simulink model "midProj"  (R2019b)
settings: Solver=VariableStepAuto  StartTime=0.0  StopTime=8  RelTol=1e-3
values from neighbouring files (symbols this model uses):
  X = 1    [midProj1102.m]    (also in midProj1103.m)
  Y = 1    [midProj1102.m]    (also in midProj1103.m)
undefined symbols (not defined in the file or in its folder): PhiDesire, PhoDesire
libraries: simulink x3
settings Model: Creator=yuhaiyang  LastModifiedBy=yuhaiyang

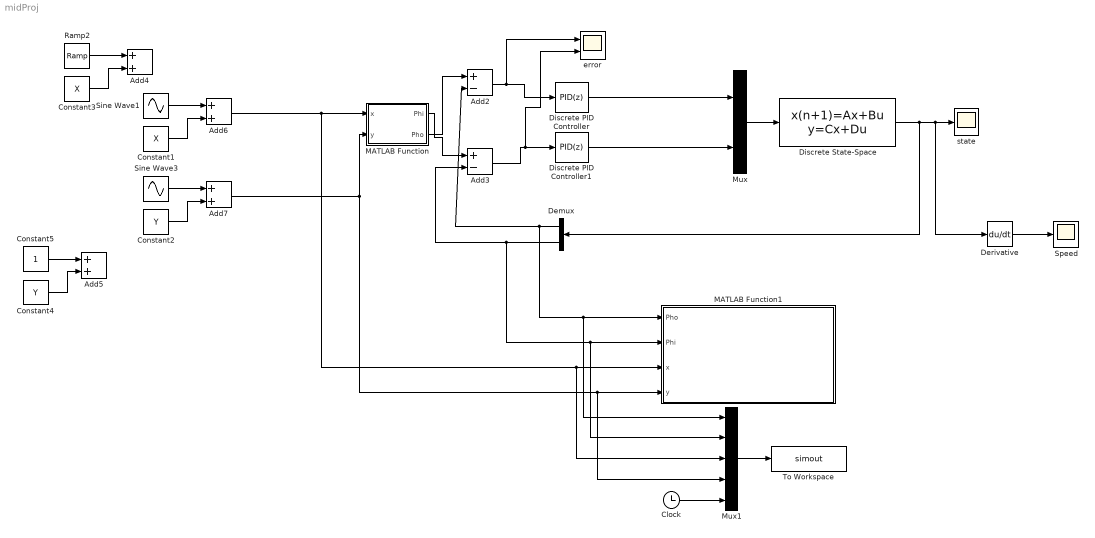
== system midProj ==
  Add2 : Sum  Inputs=+-
  Add3 : Sum  Inputs=+-
  Add{4..7} (4 alike) : Sum
  Clock : Clock
  Constant1 : Constant  Value=X
  Constant2 : Constant  Value=Y
  Constant3 : Constant  Value=X
  Constant4 : Constant  Value=Y
  Constant5 : Constant
  Demux : Demux  Outputs=2
  Derivative : Derivative
  Discrete PID Controller : simulink/Continuous/PID Controller  Controller=PID  Form=Parallel  TimeDomain=Discrete-time  SampleTime=step  IntegratorMethod=Forward Euler  FilterMethod=Forward Euler  ControllerParametersSource=internal  P=0.0451594253248729  I=0.00606949033779435  D=0.0825217736897104  UseFilter=on  N=17.4747024685303  TunerSelectOption=Transfer Function Based (PID Tuner App)  InitialConditionSource=internal  InitialConditionForIntegrator=0  InitialConditionForFilter=0  DifferentiatorICPrevScaledInput=0  ExternalReset=none  TrackingMode=off  Kt=1  LimitOutput=off  UpperSaturationLimit=inf  LowerSaturationLimit=-inf  LinearizeAsGain=off  AntiWindupMode=none  Kb=1  POutMin=[]  POutMax=[]  IOutMin=[]  IOutMax=[]  DOutMin=[]  DOutMax=[]  NOutMin=[]  NOutMax=[]  SumOutMin=[]  SumOutMax=[]  SaturationOutMin=[]  SaturationOutMax=[]  PParamMin=[]  PParamMax=[]  IParamMin=[]  IParamMax=[]  DParamMin=[]  DParamMax=[]  NParamMin=[]  NParamMax=[]  KbParamMin=[]  KbParamMax=[]  KtParamMin=[]  KtParamMax=[]  KbOutMin=[]  KbOutMax=[]  KtOutMin=[]  KtOutMax=[]  IntegratorOutMin=[]  IntegratorOutMax=[]  FilterOutMin=[]  FilterOutMax=[]  SumI1OutMin=[]  SumI1OutMax=[]  SumI2OutMin=[]  SumI2OutMax=[]  SumI3OutMin=[]  SumI3OutMax=[]  SumI4OutMin=[]  SumI4OutMax=[]  SumDOutMin=[]  SumDOutMax=[]  DifferentiatorOutMin=[]  DifferentiatorOutMax=[]  FilterDiffOutCoefMin=[]  FilterDiffOutCoefMax=[]  ReciprocalOutMin=[]  ReciprocalOutMax=[]  SumDenOutMin=[]  SumDenOutMax=[]  SumNumOutMin=[]  SumNumOutMax=[]  DivideOutMin=[]  DivideOutMax=[]  IntegratorContinuousStateAttributes=''  IntegratorStateMustResolveToSignalObject=off  IntegratorRTWStateStorageClass=Auto  FilterContinuousStateAttributes=''  FilterStateMustResolveToSignalObject=off  FilterRTWStateStorageClass=Auto  ParallelPVariant=InternalParameters  IdealPVariant=Disabled  IVariant=InternalParameters  DVariant=InternalParameters  IntegratorVariant=Discrete  SatVariant=Disabled  AWVariant=Passthrough  PCopyVariant=Disabled  TRVariant=Disabled  FdbkBlocksVariant=Forward  IdealPFdbkVariant=Disabled  SatFdbkVariant=Disabled  DerivativeFilterVariant=ForwardEulerFilter  NVariant=InternalParameters  NCopyVariant=Disabled  FilterICVariant=InternalICsFilter  IntegratorICVariant=InternalICs  ExternalResetVariant=Disabled  TRSumVariant=Passthrough  SumFdbkVariant=Disabled  SumVariant=Sum_PID
  Discrete PID Controller1 : simulink/Continuous/PID Controller  Controller=PID  Form=Parallel  TimeDomain=Discrete-time  SampleTime=step  IntegratorMethod=Forward Euler  FilterMethod=Forward Euler  ControllerParametersSource=internal  P=0.0143220434066502  I=0.00109223482739123  D=0.0463013739503765  UseFilter=on  N=12.1025626011462  TunerSelectOption=Transfer Function Based (PID Tuner App)  InitialConditionSource=internal  InitialConditionForIntegrator=0  InitialConditionForFilter=0  DifferentiatorICPrevScaledInput=0  ExternalReset=none  TrackingMode=off  Kt=1  LimitOutput=off  UpperSaturationLimit=inf  LowerSaturationLimit=-inf  LinearizeAsGain=off  AntiWindupMode=none  Kb=1  POutMin=[]  POutMax=[]  IOutMin=[]  IOutMax=[]  DOutMin=[]  DOutMax=[]  NOutMin=[]  NOutMax=[]  SumOutMin=[]  SumOutMax=[]  SaturationOutMin=[]  SaturationOutMax=[]  PParamMin=[]  PParamMax=[]  IParamMin=[]  IParamMax=[]  DParamMin=[]  DParamMax=[]  NParamMin=[]  NParamMax=[]  KbParamMin=[]  KbParamMax=[]  KtParamMin=[]  KtParamMax=[]  KbOutMin=[]  KbOutMax=[]  KtOutMin=[]  KtOutMax=[]  IntegratorOutMin=[]  IntegratorOutMax=[]  FilterOutMin=[]  FilterOutMax=[]  SumI1OutMin=[]  SumI1OutMax=[]  SumI2OutMin=[]  SumI2OutMax=[]  SumI3OutMin=[]  SumI3OutMax=[]  SumI4OutMin=[]  SumI4OutMax=[]  SumDOutMin=[]  SumDOutMax=[]  DifferentiatorOutMin=[]  DifferentiatorOutMax=[]  FilterDiffOutCoefMin=[]  FilterDiffOutCoefMax=[]  ReciprocalOutMin=[]  ReciprocalOutMax=[]  SumDenOutMin=[]  SumDenOutMax=[]  SumNumOutMin=[]  SumNumOutMax=[]  DivideOutMin=[]  DivideOutMax=[]  IntegratorContinuousStateAttributes=''  IntegratorStateMustResolveToSignalObject=off  IntegratorRTWStateStorageClass=Auto  FilterContinuousStateAttributes=''  FilterStateMustResolveToSignalObject=off  FilterRTWStateStorageClass=Auto  ParallelPVariant=InternalParameters  IdealPVariant=Disabled  IVariant=InternalParameters  DVariant=InternalParameters  IntegratorVariant=Discrete  SatVariant=Disabled  AWVariant=Passthrough  PCopyVariant=Disabled  TRVariant=Disabled  FdbkBlocksVariant=Forward  IdealPFdbkVariant=Disabled  SatFdbkVariant=Disabled  DerivativeFilterVariant=ForwardEulerFilter  NVariant=InternalParameters  NCopyVariant=Disabled  FilterICVariant=InternalICsFilter  IntegratorICVariant=InternalICs  ExternalResetVariant=Disabled  TRSumVariant=Passthrough  SumFdbkVariant=Disabled  SumVariant=Sum_PID
  Discrete State-Space : DiscreteStateSpace  A=|  B=|  C=[1,0,0,0;0,1,0,0]  D=[0,0;0,0]  InitialCondition=[PhoDesire,PhiDesire,0,0]'  SampleTime=step
      A=|
      | [1,0,step,0;
      |     0,1,0,step;
      |     0,0,1,0;
      |     0,0,0,1];
      B=|
      | [0,0;
      |     0,0;
      |     100*pi/180,0;
      |     0,100*pi/180];
  MATLAB Function : MATLAB Function  TreatAsAtomicUnit=on
  MATLAB Function1 : MATLAB Function  TreatAsAtomicUnit=on
  Mux : Mux  Inputs=2
  Mux1 : Mux  Inputs=5
  Ramp2 : simulink/Sources/Ramp  slope=0.2  start=0  InitialOutput=0
  Sine Wave1 : Sin  Frequency=0.5  SampleTime=step
  Sine Wave3 : Sin  Frequency=0.5  Phase=pi/2  SampleTime=step
  Speed : Scope
  To Workspace : ToWorkspace  VariableName=simout  SampleTime=-1
      settings: Save2DSignal=2-D array (concatenate along first dimension)
  "error " : Scope  NumInputPorts=2
  state : Scope
  wires:
  Mux/1 -> Discrete State-Space/1
  Discrete State-Space/1 -> Demux/1, Derivative/1, state/1
  Demux/1 -> Mux1/1, MATLAB Function1/1(Pho), Add2/2
  Demux/2 -> Mux1/2, MATLAB Function1/2(Phi), Add3/2
  Add2/1 -> "error "/1, Discrete PID Controller/1
  Add3/1 -> "error "/2, Discrete PID Controller1/1
  Discrete PID Controller/1 -> Mux/1
  Discrete PID Controller1/1 -> Mux/2
  Add7/1 -> MATLAB Function/2(y), Mux1/4, MATLAB Function1/4(y)
  MATLAB Function/2(Pho) -> Add2/1
  MATLAB Function/1(Phi) -> Add3/1
  Add6/1 -> Mux1/3, MATLAB Function1/3(x), MATLAB Function/1(x)
  Mux1/1 -> To Workspace/1
  Clock/1 -> Mux1/5
  Sine Wave1/1 -> Add6/1
  Constant1/1 -> Add6/2
  Sine Wave3/1 -> Add7/1
  Constant2/1 -> Add7/2
  Derivative/1 -> Speed/1
  Ramp2/1 -> Add4/1
  Constant3/1 -> Add4/2
  Constant5/1 -> Add5/1
  Constant4/1 -> Add5/2

== matlab function midProj/MATLAB Function1 ==
  data: Pho input; Phi input; x input; y input
function detectPlot(Pho,Phi,x,y)

X = 1;
Y = 1;
Z = 6;
z = 0;
axis([-1 3 -1 3,0,6])
detect(X,Y,Z,Pho,Phi);
alpha(0.25);
hold on
plot3(x,y,z,'r*')
hold on

== matlab function midProj/MATLAB Function ==
  data: x input; Phi output; y input; Pho output
function [Phi,Pho] = fcn(x,y)
z = 0;
X = 1;
Y = 1;
Z = 6;

dist = sqrt((x-X)^2+(y-Y)^2+(z-Z)^2);
Phi = acos((z-Z)/dist);

if y<Y
    Pho = atan(-(x-X)/(y-Y));
elseif y>Y
    Pho = pi+atan(-(x-X)/(y-Y));
else
    if x>X
        Pho = pi/2;
    else
        Pho = pi+pi/2;
    end
end
